simulink model "pneumaticSimscape"  (R2018b)
settings: Solver=VariableStepAuto  StartTime=0.0  StopTime=10  RelTol=1e-3
PreLoadFcn:
  | pneumaticInitialization
values from neighbouring files (symbols this model uses):
  A_pipe = 5e-4    (= 0.0005)    [pneumaticInitialization.m]
  A_piston = 0.0020    (= 0.002)    [pneumaticInitialization.m]
  delta_p = 0.6    [pneumaticInitialization.m]
  L_pipe = 1    [pneumaticInitialization.m]
  L_piston = 0.2    [pneumaticInitialization.m]
  p_init = 0.1013    [pneumaticInitialization.m]
  T_init = 293.1500    (= 293.15)    [pneumaticInitialization.m]
undefined symbols (not defined in the file or in its folder): sigbuilder_block
libraries: fl_lib x44, nesl_utility x10, SimscapeFluids_lib x1
(part 2 of 2)

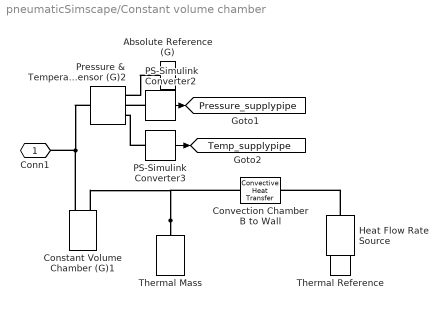
== system pneumaticSimscape/Constant volume chamber ==
  Absolute Reference (G) : fl_lib/Gas/Elements/Absolute Reference (G)
      settings: SourceProductName=Simscape  SourceProductBaseCode=SS
  Constant Volume Chamber (G)1 : fl_lib/Gas/Elements/Constant Volume Chamber (G)  volume=volume m^3  area_A=area_A m^2  p_chamber_specify=on  p_chamber_priority=High  p_chamber=p_chamber MPa  p_chamber_nominal_specify=off  p_chamber_nominal_unit=MPa  p_chamber_nominal_value=1  T_chamber_specify=off  T_chamber_priority=High  T_chamber=293.15 K  T_chamber_nominal_specify=off  T_chamber_nominal_unit=K  T_chamber_nominal_value=1  rho_chamber_specify=off  rho_chamber_priority=None  rho_chamber=1.2 kg/m^3  rho_chamber_nominal_specify=off  rho_chamber_nominal_unit=kg/m^3  rho_chamber_nominal_value=1
      settings: SourceProductName=Simscape  SourceProductBaseCode=SS
  Convection Chamber B to Wall : fl_lib/Thermal/Thermal Elements/Convective Heat Transfer  area=area m^2  heat_tr_coeff=heat_tr_coeff W/(m^2 * K)  T_specify=off  T_priority=None  T=0 K  T_nominal_specify=off  T_nominal_unit=K  T_nominal_value=1  Q_specify=off  Q_priority=None  Q=0 W  Q_nominal_specify=off  Q_nominal_unit=W  Q_nominal_value=1
  Heat Flow Rate Source : fl_lib/Thermal/Thermal Sources/Heat Flow Rate Source  heat_flow=heat_flow W
      settings: SourceProductName=Simscape  SourceProductBaseCode=SS
  PS-Simulink Converter2 : nesl_utility/PS-Simulink Converter  PhysicalDomain=network_engine_domain  SubClassName=ps_output  LeftPortType=input  RightPortType=output  PseudoPeriodic=off  Frequencies=[]  Unit=1  AffineConversion=off
  PS-Simulink Converter3 : nesl_utility/PS-Simulink Converter  PhysicalDomain=network_engine_domain  SubClassName=ps_output  LeftPortType=input  RightPortType=output  PseudoPeriodic=off  Frequencies=[]  Unit=1  AffineConversion=off
  Pressure & Temperature Sensor (G)2 : fl_lib/Gas/Sensors/Pressure & Temperature Sensor (G)
      settings: SourceProductName=Simscape  SourceProductBaseCode=SS
  Thermal Mass : fl_lib/Thermal/Thermal Elements/Thermal Mass  mass=0.214 kg  sp_heat=840 J/kg/K  T_specify=on  T_priority=High  T=293.15 K  T_nominal_specify=off  T_nominal_unit=K  T_nominal_value=1  Q_specify=off  Q_priority=None  Q=0 W  Q_nominal_specify=off  Q_nominal_unit=W  Q_nominal_value=1
  Thermal Reference : fl_lib/Thermal/Thermal Elements/Thermal Reference
  Conn1 : PMIOPort  Side=Left
  tag scope: Pressure_supplypipe=global, Temp_supplypipe=global
  wires:
  PS-Simulink Converter3/1 -> [Temp_supplypipe]
  PS-Simulink Converter2/1 -> [Pressure_supplypipe]
  connections:
  Thermal Reference/LConn1 -- Heat Flow Rate Source/RConn1
  Constant Volume Chamber (G)1/LConn1 -- Pressure & Temperature Sensor (G)2/LConn1 -- Conn1/RConn1
  Thermal Mass/LConn1 -- Convection Chamber B to Wall/RConn1 -- Constant Volume Chamber (G)1/LConn2
  Heat Flow Rate Source/LConn1 -- Convection Chamber B to Wall/LConn1
  PS-Simulink Converter2/LConn1 -- Pressure & Temperature Sensor (G)2/RConn2
  Absolute Reference (G)/LConn1 -- Pressure & Temperature Sensor (G)2/RConn1
  PS-Simulink Converter3/LConn1 -- Pressure & Temperature Sensor (G)2/RConn3

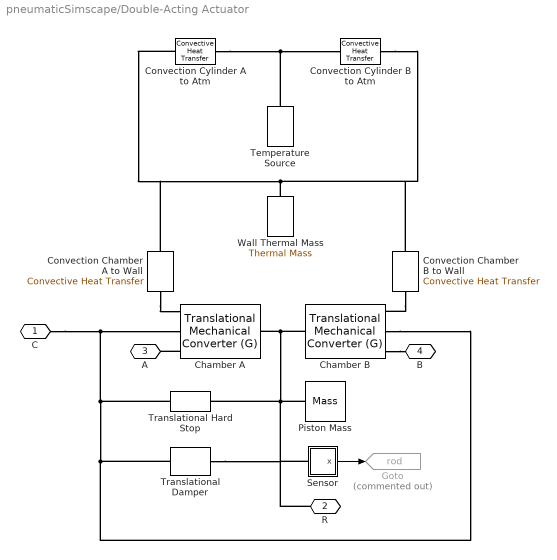
== system pneumaticSimscape/Double-Acting Actuator ==
  Chamber A : fl_lib/Gas/Elements/Translational Mechanical Converter (G)  mech_orientation=1  interface_area=A_piston m^2  length_init=x_init m  dead_volume=0.1 * A_piston * x_max m^3  area_A=A_port m^2  environment_spec=1  environment_pressure=0.101325 MPa  p_converter_specify=on  p_converter_priority=High  p_converter=p_init MPa  p_converter_nominal_specify=off  p_converter_nominal_unit=MPa  p_converter_nominal_value=1  T_converter_specify=on  T_converter_priority=High  T_converter=T_init K  T_converter_nominal_specify=off  T_converter_nominal_unit=K  T_converter_nominal_value=1  rho_converter_specify=off  rho_converter_priority=None  rho_converter=1.2 kg/m^3  rho_converter_nominal_specify=off  rho_converter_nominal_unit=kg/m^3  rho_converter_nominal_value=1
      settings: SourceProductName=Simscape  SourceProductBaseCode=SS
  Chamber B : fl_lib/Gas/Elements/Translational Mechanical Converter (G)  mech_orientation=-1  interface_area=A_piston m^2  length_init=- x_max + x_init m  dead_volume=0.1 * A_piston * x_max m^3  area_A=A_port m^2  environment_spec=1  environment_pressure=0.101325 MPa  p_converter_specify=on  p_converter_priority=High  p_converter=p_init MPa  p_converter_nominal_specify=off  p_converter_nominal_unit=MPa  p_converter_nominal_value=1  T_converter_specify=on  T_converter_priority=High  T_converter=T_init K  T_converter_nominal_specify=off  T_converter_nominal_unit=K  T_converter_nominal_value=1  rho_converter_specify=off  rho_converter_priority=None  rho_converter=1.2 kg/m^3  rho_converter_nominal_specify=off  rho_converter_nominal_unit=kg/m^3  rho_converter_nominal_value=1
      settings: SourceProductName=Simscape  SourceProductBaseCode=SS
  Convection Chamber A to Wall : fl_lib/Thermal/Thermal Elements/Convective Heat Transfer  area=2*A_piston + sqrt(pi*A_piston)*x_max m^2  heat_tr_coeff=heat_coeff W/(m^2 * K)  T_specify=off  T_priority=None  T=0 K  T_nominal_specify=off  T_nominal_unit=K  T_nominal_value=1  Q_specify=off  Q_priority=None  Q=0 W  Q_nominal_specify=off  Q_nominal_unit=W  Q_nominal_value=1
  Convection Chamber B to Wall : fl_lib/Thermal/Thermal Elements/Convective Heat Transfer  area=2*A_piston + sqrt(pi*A_piston)*x_max m^2  heat_tr_coeff=heat_coeff W/(m^2 * K)  T_specify=off  T_priority=None  T=0 K  T_nominal_specify=off  T_nominal_unit=K  T_nominal_value=1  Q_specify=off  Q_priority=None  Q=0 W  Q_nominal_specify=off  Q_nominal_unit=W  Q_nominal_value=1
  Convection Cylinder A to Atm : fl_lib/Thermal/Thermal Elements/Convective Heat Transfer  area=2*A_piston + sqrt(pi*A_piston)*L_piston m^2  heat_tr_coeff=20 W/(m^2 * K)  T_specify=off  T_priority=None  T=0 K  T_nominal_specify=off  T_nominal_unit=K  T_nominal_value=1  Q_specify=off  Q_priority=None  Q=0 W  Q_nominal_specify=off  Q_nominal_unit=W  Q_nominal_value=1
  Convection Cylinder B to Atm : fl_lib/Thermal/Thermal Elements/Convective Heat Transfer  area=2*A_piston + sqrt(pi*A_piston)*L_piston m^2  heat_tr_coeff=20 W/(m^2 * K)  T_specify=off  T_priority=None  T=0 K  T_nominal_specify=off  T_nominal_unit=K  T_nominal_value=1  Q_specify=off  Q_priority=None  Q=0 W  Q_nominal_specify=off  Q_nominal_unit=W  Q_nominal_value=1
  Goto : Goto  Commented=on  GotoTag=rod  TagVisibility=global
  Piston Mass : fl_lib/Mechanical/Translational Elements/Mass  mass=M_piston kg  v_specify=off  v_priority=High  v=0 m/s  v_nominal_specify=off  v_nominal_unit=m/s  v_nominal_value=1  f_specify=off  f_priority=None  f=0 N  f_nominal_specify=off  f_nominal_unit=N  f_nominal_value=1
  Sensor : Subsystem
      mask Display: disp('S')
  Temperature Source : fl_lib/Thermal/Thermal Sources/Temperature Source  temperature=T_atm K
      settings: SourceProductName=Simscape
  Translational Damper : fl_lib/Mechanical/Translational Elements/Translational Damper  D=damp_mech N/(m/s)  v_specify=off  v_priority=None  v=0 m/s  v_nominal_specify=off  v_nominal_unit=m/s  v_nominal_value=1  f_specify=off  f_priority=None  f=0 N  f_nominal_specify=off  f_nominal_unit=N  f_nominal_value=1
  Translational Hard Stop : fl_lib/Mechanical/Translational Elements/Translational Hard Stop  upper_bnd=x_max m  lower_bnd=0 m  stiff_up=stiff_hard_stop N/m  stiff_low=stiff_hard_stop N/m  D_up=damp_hard_stop N/(m/s)  D_low=damp_hard_stop N/(m/s)  model=3  transition=0.1 mm  v_specify=off  v_priority=None  v=0 m/s  v_nominal_specify=off  v_nominal_unit=m/s  v_nominal_value=1  f_specify=off  f_priority=None  f=0 N  f_nominal_specify=off  f_nominal_unit=N  f_nominal_value=1  x_specify=on  x_priority=High  x=x_init m  x_nominal_specify=off  x_nominal_unit=m  x_nominal_value=1
  Wall Thermal Mass : fl_lib/Thermal/Thermal Elements/Thermal Mass  mass=M_actuator kg  sp_heat=cp J/kg/K  T_specify=on  T_priority=High  T=T_init K  T_nominal_specify=off  T_nominal_unit=K  T_nominal_value=1  Q_specify=off  Q_priority=None  Q=0 W  Q_nominal_specify=off  Q_nominal_unit=W  Q_nominal_value=1
  C : PMIOPort  Side=Left
  R : PMIOPort  Port=2  Side=Right
  A : PMIOPort  Port=3  Side=Left
  B : PMIOPort  Port=4  Side=Right
  wires:
  Sensor/1(x) -> Goto/1
  connections:
  Chamber B/RConn1 -- R/RConn1 -- Sensor/LConn1 -- Translational Damper/LConn1 -- Piston Mass/LConn1 -- Translational Hard Stop/LConn1 -- Chamber A/RConn1
  Convection Cylinder A to Atm/LConn1 -- Convection Chamber A to Wall/RConn1 -- Wall Thermal Mass/LConn1 -- Convection Cylinder B to Atm/LConn1 -- Convection Chamber B to Wall/RConn1
  Translational Hard Stop/RConn1 -- Chamber B/LConn2 -- Translational Damper/RConn1 -- C/RConn1 -- Chamber A/LConn2
  Chamber A/LConn1 -- A/RConn1
  Chamber B/LConn1 -- B/RConn1
  Convection Chamber A to Wall/LConn1 -- Chamber A/LConn3
  Convection Chamber B to Wall/LConn1 -- Chamber B/LConn3
  Convection Cylinder A to Atm/RConn1 -- Temperature Source/LConn1 -- Convection Cylinder B to Atm/RConn1

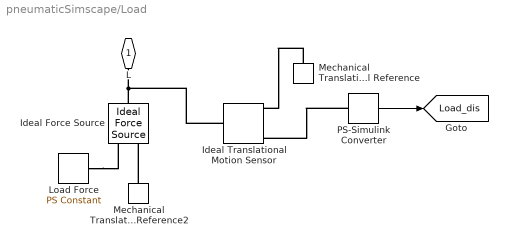
== system pneumaticSimscape/Load ==
  Ideal Force Source : fl_lib/Mechanical/Mechanical Sources/Ideal Force Source
  Ideal Translational Motion Sensor : fl_lib/Mechanical/Mechanical Sensors/Ideal Translational Motion Sensor  offset=0 m
  Load Force : fl_lib/Physical Signals/Sources/PS Constant  constant=-500
  Mechanical Translational Reference : fl_lib/Mechanical/Translational Elements/Mechanical Translational Reference
  Mechanical Translational Reference2 : fl_lib/Mechanical/Translational Elements/Mechanical Translational Reference
  PS-Simulink Converter : nesl_utility/PS-Simulink Converter  PhysicalDomain=network_engine_domain  SubClassName=ps_output  LeftPortType=input  RightPortType=output  PseudoPeriodic=off  Frequencies=[]  Unit=m  AffineConversion=off
  L : PMIOPort  Side=Right
  tag scope: Load_dis=global
  wires:
  PS-Simulink Converter/1 -> [Load_dis]
  connections:
  Load Force/RConn1 -- Ideal Force Source/RConn1
  Mechanical Translational Reference2/LConn1 -- Ideal Force Source/RConn2
  Ideal Force Source/LConn1 -- Ideal Translational Motion Sensor/LConn1 -- L/RConn1
  PS-Simulink Converter/LConn1 -- Ideal Translational Motion Sensor/RConn3
  Mechanical Translational Reference/LConn1 -- Ideal Translational Motion Sensor/RConn1

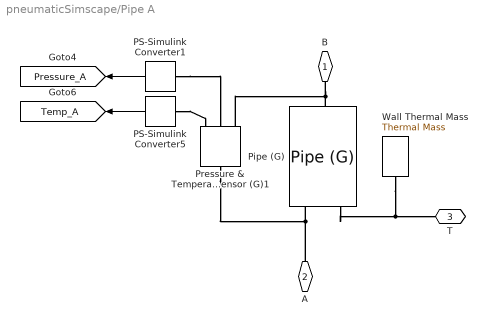
== system pneumaticSimscape/Pipe A ==
  PS-Simulink Converter1 : nesl_utility/PS-Simulink Converter  PhysicalDomain=network_engine_domain  SubClassName=ps_output  LeftPortType=input  RightPortType=output  PseudoPeriodic=off  Frequencies=[]  Unit=1  AffineConversion=off
  PS-Simulink Converter5 : nesl_utility/PS-Simulink Converter  PhysicalDomain=network_engine_domain  SubClassName=ps_output  LeftPortType=input  RightPortType=output  PseudoPeriodic=off  Frequencies=[]  Unit=1  AffineConversion=off
  Pipe (G) : fl_lib/Gas/Elements/Pipe (G)  length=L_pipe m  area=A_pipe m^2  Dh=2*sqrt(A_pipe/pi) m  length_add=0.1 * L_pipe m  roughness=15e-6 m  Re_lam=2000  Re_tur=4000  shape_factor=64  Nu_lam=3.66  p_pipe_specify=on  p_pipe_priority=High  p_pipe=p_init MPa  p_pipe_nominal_specify=off  p_pipe_nominal_unit=MPa  p_pipe_nominal_value=1  T_pipe_specify=on  T_pipe_priority=High  T_pipe=T_init K  T_pipe_nominal_specify=off  T_pipe_nominal_unit=K  T_pipe_nominal_value=1  rho_pipe_specify=off  rho_pipe_priority=None  rho_pipe=1.2 kg/m^3  rho_pipe_nominal_specify=off  rho_pipe_nominal_unit=kg/m^3  rho_pipe_nominal_value=1
      settings: SourceProductName=Simscape  SourceProductBaseCode=SS
  Pressure & Temperature Sensor (G)1 : fl_lib/Gas/Sensors/Pressure & Temperature Sensor (G)
      settings: SourceProductName=Simscape  SourceProductBaseCode=SS
  Wall Thermal Mass : fl_lib/Thermal/Thermal Elements/Thermal Mass  mass=rho_wall * A_pipe * L_pipe kg  sp_heat=cp_wall J/kg/K  T_specify=on  T_priority=High  T=T_init K  T_nominal_specify=off  T_nominal_unit=K  T_nominal_value=1  Q_specify=off  Q_priority=None  Q=0 W  Q_nominal_specify=off  Q_nominal_unit=W  Q_nominal_value=1
  B : PMIOPort  Side=Right
  A : PMIOPort  Port=2  Side=Left
  T : PMIOPort  Port=3  Side=Left
  tag scope: Pressure_A=global, Temp_A=global
  wires:
  PS-Simulink Converter5/1 -> [Temp_A]
  PS-Simulink Converter1/1 -> [Pressure_A]
  connections:
  Pipe (G)/RConn1 -- Pressure & Temperature Sensor (G)1/RConn1 -- B/RConn1
  A/RConn1 -- Pressure & Temperature Sensor (G)1/LConn1 -- Pipe (G)/LConn1
  Pipe (G)/LConn2 -- Wall Thermal Mass/LConn1 -- T/RConn1
  PS-Simulink Converter5/LConn1 -- Pressure & Temperature Sensor (G)1/RConn3
  PS-Simulink Converter1/LConn1 -- Pressure & Temperature Sensor (G)1/RConn2

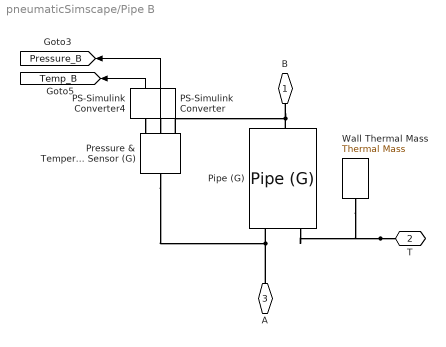
== system pneumaticSimscape/Pipe B ==
  PS-Simulink Converter : nesl_utility/PS-Simulink Converter  PhysicalDomain=network_engine_domain  SubClassName=ps_output  LeftPortType=input  RightPortType=output  PseudoPeriodic=off  Frequencies=[]  Unit=1  AffineConversion=off
  PS-Simulink Converter4 : nesl_utility/PS-Simulink Converter  PhysicalDomain=network_engine_domain  SubClassName=ps_output  LeftPortType=input  RightPortType=output  PseudoPeriodic=off  Frequencies=[]  Unit=1  AffineConversion=off
  Pipe (G) : fl_lib/Gas/Elements/Pipe (G)  length=L_pipe m  area=A_pipe m^2  Dh=2*sqrt(A_pipe/pi) m  length_add=0.1 * L_pipe m  roughness=15e-6 m  Re_lam=2000  Re_tur=4000  shape_factor=64  Nu_lam=3.66  p_pipe_specify=on  p_pipe_priority=High  p_pipe=p_init MPa  p_pipe_nominal_specify=off  p_pipe_nominal_unit=MPa  p_pipe_nominal_value=1  T_pipe_specify=on  T_pipe_priority=High  T_pipe=T_init K  T_pipe_nominal_specify=off  T_pipe_nominal_unit=K  T_pipe_nominal_value=1  rho_pipe_specify=off  rho_pipe_priority=None  rho_pipe=1.2 kg/m^3  rho_pipe_nominal_specify=off  rho_pipe_nominal_unit=kg/m^3  rho_pipe_nominal_value=1
      settings: SourceProductName=Simscape  SourceProductBaseCode=SS
  Pressure & Temperature Sensor (G) : fl_lib/Gas/Sensors/Pressure & Temperature Sensor (G)
      settings: SourceProductName=Simscape  SourceProductBaseCode=SS
  Wall Thermal Mass : fl_lib/Thermal/Thermal Elements/Thermal Mass  mass=rho_wall * A_pipe * L_pipe kg  sp_heat=cp_wall J/kg/K  T_specify=on  T_priority=High  T=T_init K  T_nominal_specify=off  T_nominal_unit=K  T_nominal_value=1  Q_specify=off  Q_priority=None  Q=0 W  Q_nominal_specify=off  Q_nominal_unit=W  Q_nominal_value=1
  B : PMIOPort  Side=Right
  T : PMIOPort  Port=2  Side=Left
  A : PMIOPort  Port=3  Side=Left
  tag scope: Pressure_B=global, Temp_B=global
  wires:
  PS-Simulink Converter4/1 -> [Temp_B]
  PS-Simulink Converter/1 -> [Pressure_B]
  connections:
  T/RConn1 -- Wall Thermal Mass/LConn1 -- Pipe (G)/LConn2
  A/RConn1 -- Pressure & Temperature Sensor (G)/LConn1 -- Pipe (G)/LConn1
  Pipe (G)/RConn1 -- Pressure & Temperature Sensor (G)/RConn1 -- B/RConn1
  PS-Simulink Converter4/LConn1 -- Pressure & Temperature Sensor (G)/RConn3
  PS-Simulink Converter/LConn1 -- Pressure & Temperature Sensor (G)/RConn2

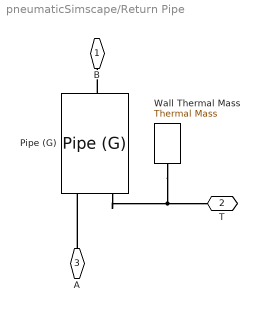
== system pneumaticSimscape/Return Pipe ==
  Pipe (G) : fl_lib/Gas/Elements/Pipe (G)  length=L_pipe m  area=A_pipe m^2  Dh=2*sqrt(A_pipe/pi) m  length_add=0.1 * L_pipe m  roughness=15e-6 m  Re_lam=2000  Re_tur=4000  shape_factor=64  Nu_lam=3.66  p_pipe_specify=on  p_pipe_priority=High  p_pipe=p_init MPa  p_pipe_nominal_specify=off  p_pipe_nominal_unit=MPa  p_pipe_nominal_value=1  T_pipe_specify=on  T_pipe_priority=High  T_pipe=T_init K  T_pipe_nominal_specify=off  T_pipe_nominal_unit=K  T_pipe_nominal_value=1  rho_pipe_specify=off  rho_pipe_priority=None  rho_pipe=1.2 kg/m^3  rho_pipe_nominal_specify=off  rho_pipe_nominal_unit=kg/m^3  rho_pipe_nominal_value=1
      settings: SourceProductName=Simscape  SourceProductBaseCode=SS
  Wall Thermal Mass : fl_lib/Thermal/Thermal Elements/Thermal Mass  mass=rho_wall * A_pipe * L_pipe kg  sp_heat=cp_wall J/kg/K  T_specify=on  T_priority=High  T=T_init K  T_nominal_specify=off  T_nominal_unit=K  T_nominal_value=1  Q_specify=off  Q_priority=None  Q=0 W  Q_nominal_specify=off  Q_nominal_unit=W  Q_nominal_value=1
  B : PMIOPort  Side=Right
  T : PMIOPort  Port=2  Side=Left
  A : PMIOPort  Port=3  Side=Left
  connections:
  Pipe (G)/RConn1 -- B/RConn1
  A/RConn1 -- Pipe (G)/LConn1
  Pipe (G)/LConn2 -- Wall Thermal Mass/LConn1 -- T/RConn1

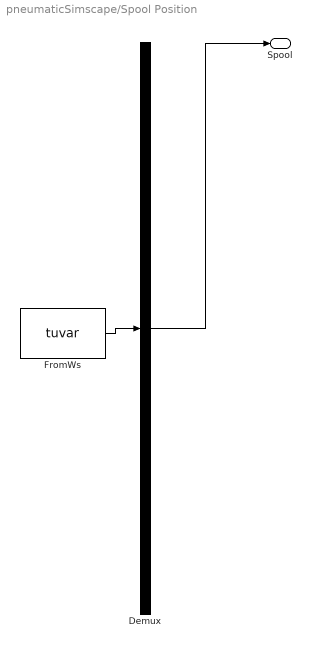
== system pneumaticSimscape/Spool Position ==
  Demux : Demux  Tag=STV Demux  Outputs=1
  FromWs : FromWorkspace  Tag=STV FromWs  VariableName=tuvar  SampleTime=0
      SigBuilderData=|
      | common.afterFinalStr = 'Extrapolate'
      | common.sampleTime = 0
      | dataSet.timeRange = [0 10]
      | dataSet.name = 'Group 1'
      | sbobj.Groups.Name = 'Group 1'
      | sbobj.Groups.Signals.Name = 'Spool'
      | sbobj.Groups.Signals.XData = [0 1 1.2 3.8 4 6 6.2 8.8 9 10]
      | sbobj.Groups.Signals.YData = [0 0 5 5 0 0 -5 -5 0 0]
  Spool : Outport  Tag=STV Outport
  wires:
  Demux/1 -> Spool/1
  FromWs/1 -> Demux/1

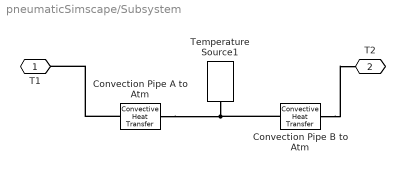
== system pneumaticSimscape/Subsystem ==
  Convection Pipe A to Atm : fl_lib/Thermal/Thermal Elements/Convective Heat Transfer  area=2*sqrt(pi*A_pipe) * L_pipe m^2  heat_tr_coeff=20 W/(m^2 * K)  T_specify=off  T_priority=None  T=0 K  T_nominal_specify=off  T_nominal_unit=K  T_nominal_value=1  Q_specify=off  Q_priority=None  Q=0 W  Q_nominal_specify=off  Q_nominal_unit=W  Q_nominal_value=1
  Convection Pipe B to Atm : fl_lib/Thermal/Thermal Elements/Convective Heat Transfer  area=2*sqrt(pi*A_pipe) * L_pipe m^2  heat_tr_coeff=20 W/(m^2 * K)  T_specify=off  T_priority=None  T=0 K  T_nominal_specify=off  T_nominal_unit=K  T_nominal_value=1  Q_specify=off  Q_priority=None  Q=0 W  Q_nominal_specify=off  Q_nominal_unit=W  Q_nominal_value=1
  Temperature Source1 : fl_lib/Thermal/Thermal Sources/Temperature Source  temperature=T_atm K
      settings: SourceProductName=Simscape
  T1 : PMIOPort  Side=Left
  T2 : PMIOPort  Port=2  Side=Left
  connections:
  Convection Pipe B to Atm/RConn1 -- Temperature Source1/LConn1 -- Convection Pipe A to Atm/RConn1
  Convection Pipe A to Atm/LConn1 -- T1/RConn1
  Convection Pipe B to Atm/LConn1 -- T2/RConn1

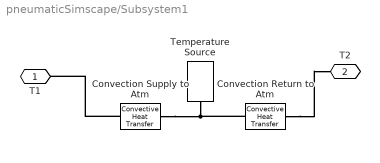
== system pneumaticSimscape/Subsystem1 ==
  Convection Return to Atm : fl_lib/Thermal/Thermal Elements/Convective Heat Transfer  area=2*sqrt(pi*A_pipe) * L_pipe m^2  heat_tr_coeff=20 W/(m^2 * K)  T_specify=off  T_priority=None  T=0 K  T_nominal_specify=off  T_nominal_unit=K  T_nominal_value=1  Q_specify=off  Q_priority=None  Q=0 W  Q_nominal_specify=off  Q_nominal_unit=W  Q_nominal_value=1
  Convection Supply to Atm : fl_lib/Thermal/Thermal Elements/Convective Heat Transfer  area=2*sqrt(pi*A_pipe) * L_pipe m^2  heat_tr_coeff=20 W/(m^2 * K)  T_specify=off  T_priority=None  T=0 K  T_nominal_specify=off  T_nominal_unit=K  T_nominal_value=1  Q_specify=off  Q_priority=None  Q=0 W  Q_nominal_specify=off  Q_nominal_unit=W  Q_nominal_value=1
  Temperature Source : fl_lib/Thermal/Thermal Sources/Temperature Source  temperature=T_atm K
      settings: SourceProductName=Simscape
  T1 : PMIOPort  Side=Left
  T2 : PMIOPort  Port=2  Side=Left
  connections:
  Convection Return to Atm/RConn1 -- Temperature Source/LConn1 -- Convection Supply to Atm/RConn1
  Convection Supply to Atm/LConn1 -- T1/RConn1
  Convection Return to Atm/LConn1 -- T2/RConn1

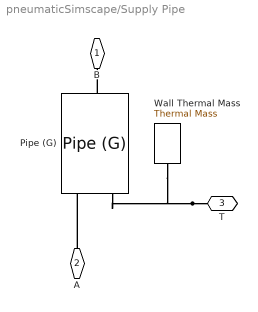
== system pneumaticSimscape/Supply Pipe ==
  Pipe (G) : fl_lib/Gas/Elements/Pipe (G)  length=L_pipe m  area=A_pipe m^2  Dh=2*sqrt(A_pipe/pi) m  length_add=0.1 * L_pipe m  roughness=15e-6 m  Re_lam=2000  Re_tur=4000  shape_factor=64  Nu_lam=3.66  p_pipe_specify=on  p_pipe_priority=High  p_pipe=p_init MPa  p_pipe_nominal_specify=off  p_pipe_nominal_unit=MPa  p_pipe_nominal_value=1  T_pipe_specify=on  T_pipe_priority=High  T_pipe=T_init K  T_pipe_nominal_specify=off  T_pipe_nominal_unit=K  T_pipe_nominal_value=1  rho_pipe_specify=off  rho_pipe_priority=None  rho_pipe=1.2 kg/m^3  rho_pipe_nominal_specify=off  rho_pipe_nominal_unit=kg/m^3  rho_pipe_nominal_value=1
      settings: SourceProductName=Simscape  SourceProductBaseCode=SS
  Wall Thermal Mass : fl_lib/Thermal/Thermal Elements/Thermal Mass  mass=rho_wall * A_pipe * L_pipe kg  sp_heat=cp_wall J/kg/K  T_specify=on  T_priority=High  T=T_init K  T_nominal_specify=off  T_nominal_unit=K  T_nominal_value=1  Q_specify=off  Q_priority=None  Q=0 W  Q_nominal_specify=off  Q_nominal_unit=W  Q_nominal_value=1
  B : PMIOPort  Side=Right
  A : PMIOPort  Port=2  Side=Left
  T : PMIOPort  Port=3  Side=Left
  connections:
  T/RConn1 -- Wall Thermal Mass/LConn1 -- Pipe (G)/LConn2
  A/RConn1 -- Pipe (G)/LConn1
  Pipe (G)/RConn1 -- B/RConn1

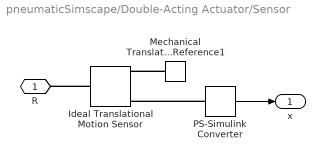
== system pneumaticSimscape/Double-Acting Actuator/Sensor ==
  Ideal Translational Motion Sensor : fl_lib/Mechanical/Mechanical Sensors/Ideal Translational Motion Sensor  offset=0 m
  Mechanical Translational Reference1 : fl_lib/Mechanical/Translational Elements/Mechanical Translational Reference
  PS-Simulink Converter : nesl_utility/PS-Simulink Converter  PhysicalDomain=network_engine_domain  SubClassName=ps_output  LeftPortType=input  RightPortType=output  PseudoPeriodic=off  Frequencies=[]  Unit=m  AffineConversion=off
  R : PMIOPort  Side=Left
  x : Outport
  wires:
  PS-Simulink Converter/1 -> x/1
  connections:
  Mechanical Translational Reference1/LConn1 -- Ideal Translational Motion Sensor/RConn1
  Ideal Translational Motion Sensor/LConn1 -- R/RConn1
  PS-Simulink Converter/LConn1 -- Ideal Translational Motion Sensor/RConn3
